simulink model "receiveAPT_RTLSDR"  (R2017a)
settings: Solver=VariableStepAuto  StartTime=0.0  StopTime=150  RelTol=1e-3
undefined symbols (not defined in the file or in its folder): designMultirateFIR
libraries: dspmathops x1, dspsigops x1, dsparch4 x1, dspmlti4 x1, sdrrlib x1
settings Model: Creator=kelnhofer  LastModifiedBy=prust

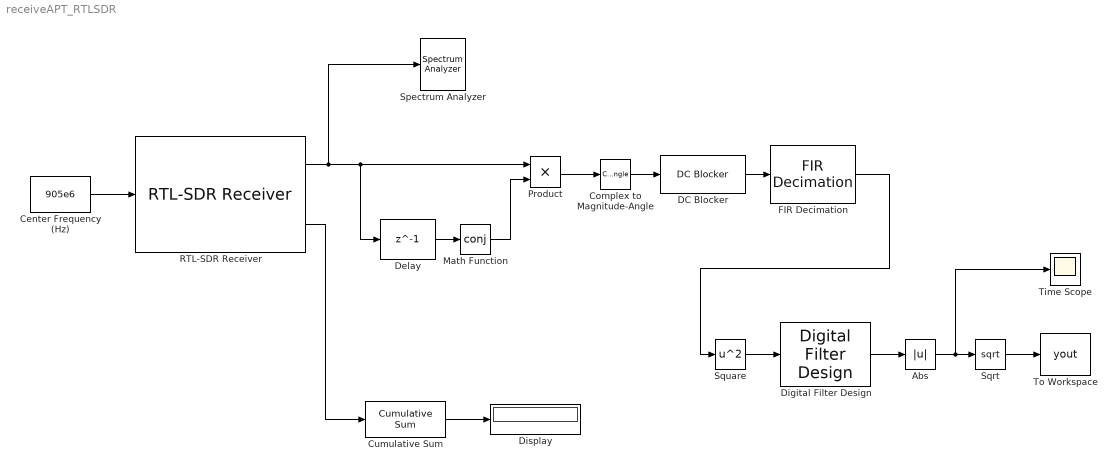
== system receiveAPT_RTLSDR ==
  Abs : Abs
  Center Frequency (Hz) : Constant  Value=905e6
  Complex to Magnitude-Angle : ComplexToMagnitudeAngle  Output=Angle
  Cumulative Sum : dspmathops/Cumulative Sum  dim=Channels (running sum)  InputProcessing=Columns as channels (frame based)  reset_popup=None  outputDataTypeStr=Inherit: Same as accumulator  outputLastDataTypeStr=Inherit: Same as accumulator  outputMin=[]  outputMax=[]  roundingMode=Floor  overflowMode=off
      settings: SourceProductName=DSP System Toolbox
  DC Blocker : dspsigops/DC Blocker  Algorithm=IIR  NormalizedBandwidth=0.001  Length=50  Order=6  SimulateUsing=Code generation
      settings: SourceProductName=DSP System Toolbox  SourceProductBaseCode=DS
  Delay : Delay  DelayLength=1  InputProcessing=Columns as channels (frame based)
  Digital Filter Design : dsparch4/Digital Filter Design  mwdsp_browser_bugfix_var=off
  Display : Display
  FIR Decimation : dspmlti4/FIR Decimation  FilterSource=Auto  h=designMultirateFIR(1,2)  D=10  filtStruct=Direct form  FilterObject=FDECIM  InputProcessing=Columns as channels (frame based)  framing=Enforce single-rate processing  inputOffset=0  outputBufInitCond=0  roundingMode=Floor  overflowMode=off  firstCoeffDataTypeStr=Inherit: Same word length as input  firstCoeffMin=[]  firstCoeffMax=[]  firstCoeffLastDataTypeStr=Inherit: Same word length as input  outputDataTypeStr=Inherit: Same as accumulator  outputMin=[]  outputMax=[]  outputLastDataTypeStr=Inherit: Same as accumulator
  Math Function : Math  Operator=conj  SaturateOnIntegerOverflow=on
  Product : Product
  RTL-SDR Receiver : sdrrlib/RTL-SDR Receiver  SourceLibraryInfo="This block requires <a href=\"http://www.mathworks.com/hardware-support/rtl-sdr.html\">Communications System Toolbox Support Package for RTL-SDR Radio</a>"  sobjType=sdrr.internal.SDRRTLReceiverSL  IPAddress=0  dataUDPPort=-1  ctrlUDPPort=-1  subDeviceList=nosubdev  sdrBlockType=SDRBlockTypeSLT.SDRRxBlock  requester=UNUSED_BY_SFCN  sdrExecutionMode=SDRExecutionModeSLT.ExecModeHW  LostSamplesOutputPort=on  OutputDataType=double  FrameLength=1000  EnableBurstMode=off  NumFramesInBurst=20  BypassUserLogic=off  DecimatorSelect=DDC decimator  SourceSelect=RF data  SineAmplitude=16000  EnableInternalClock=off  BypassIQBalance=off  CenterFrequency=102.5e6  IFBandwidth=40e6  ADCRateSource=Dialog  ADCRate=240e3  CenterFrequencySource=Input port  GainSource=Dialog  IntermediateFrequency=0  Gain=40  DecimationFactorSource=Dialog  DecimationFactor=512  RFFrequencyIsTunable=logical(1)  SampleTime=(1000)/(240e3)  IFBandwidthSource=Dialog  SineFrequency=30000  BypassDCBlockingFilter=off  IntermediateFrequencySource=Dialog  IQBalanceCoefficients=64  SkipAllHardwareResetAndInitialization=off  EnableIQCalibrationTable=on  CacheIQCalibrationTable=off  EnableOffsetTuning=off  EnableRTLAGC=off  EnableTestMode=off  EnableTunerAGC=off  FrequencyCorrectionSource=Dialog  FrequencyCorrection=0  NumMLBuffers=128  NumUSBBuffers=16  LatencyOutputPort=off  RTLCrystalFrequency=28800000  TunerCrystalFrequency=28800000
      settings: SourceProductName=Communications System Toolbox Support Package for RTL-SDR Radio  SourceProductBaseCode=RTLSDR
  Spectrum Analyzer : SpectrumAnalyzer
  Sqrt : Sqrt  SaturateOnIntegerOverflow=on
  Square : Math  Operator=square  SaturateOnIntegerOverflow=on
  Time Scope : Scope
  To Workspace : ToWorkspace  VariableName=yout  SampleTime=-1
      settings: Save2DSignal=2-D array (concatenate along first dimension)
  wires:
  RTL-SDR Receiver/1 -> Spectrum Analyzer/1, Product/1, Delay/1
  Delay/1 -> Math Function/1
  Math Function/1 -> Product/2
  Product/1 -> Complex to Magnitude-Angle/1
  Complex to Magnitude-Angle/1 -> DC Blocker/1
  Center Frequency (Hz)/1 -> RTL-SDR Receiver/1
  Square/1 -> Digital Filter Design/1
  Sqrt/1 -> To Workspace/1
  RTL-SDR Receiver/2 -> Cumulative Sum/1
  Cumulative Sum/1 -> Display/1
  FIR Decimation/1 -> Square/1
  Digital Filter Design/1 -> Abs/1
  Abs/1 -> Time Scope/1, Sqrt/1
  DC Blocker/1 -> FIR Decimation/1
